simulink model "LAB_03_3_OCT_SIM_EUL"  (R2022b)
settings: Solver=FixedStepAuto  StartTime=0.0  StopTime=100.0  FixedStep=0.1  RelTol=1e-3
values from neighbouring files (symbols this model uses):
  om_x0 = 0.45    [LAB_03_3_OCT_MAT_EUL.m]    (also in LAB_03_3_OCT_MAT_EUL_2_VERIFICATION.m = 6.28318530718; LAB_03_3_OCT_MAT_EUL_DOUBLESPIN.m = 1e-06; LAB_03_3_OCT_MAT_EUL_SPINAXIS.m = 0.1; LAB_03_3_OCT_MAT_EUL_VECT.m)
  om_y0 = 0.52    [LAB_03_3_OCT_MAT_EUL.m]    (also in LAB_03_3_OCT_MAT_EUL_2_VERIFICATION.m = 0; LAB_03_3_OCT_MAT_EUL_DOUBLESPIN.m = 1e-06; LAB_03_3_OCT_MAT_EUL_SPINAXIS.m = 6.28318530718; LAB_03_3_OCT_MAT_EUL_VECT.m)
  om_z0 = 0.55    [LAB_03_3_OCT_MAT_EUL.m]    (also in LAB_03_3_OCT_MAT_EUL_2_VERIFICATION.m = 0; LAB_03_3_OCT_MAT_EUL_DOUBLESPIN.m = 0.02; LAB_03_3_OCT_MAT_EUL_SPINAXIS.m = 0.1; LAB_03_3_OCT_MAT_EUL_VECT.m)
settings Model: Creator=maria  LastModifiedBy=maria

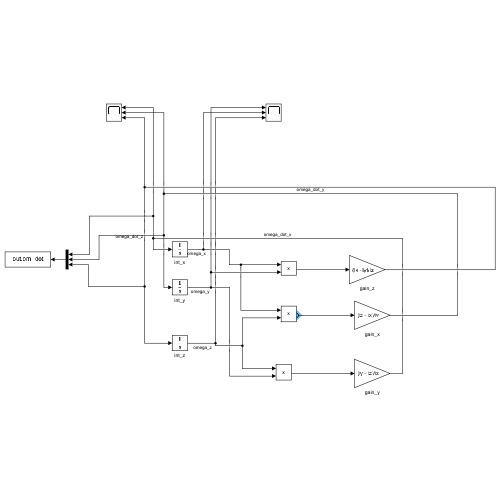
[thumbnail: Simulink's stored preview of the top-level diagram]
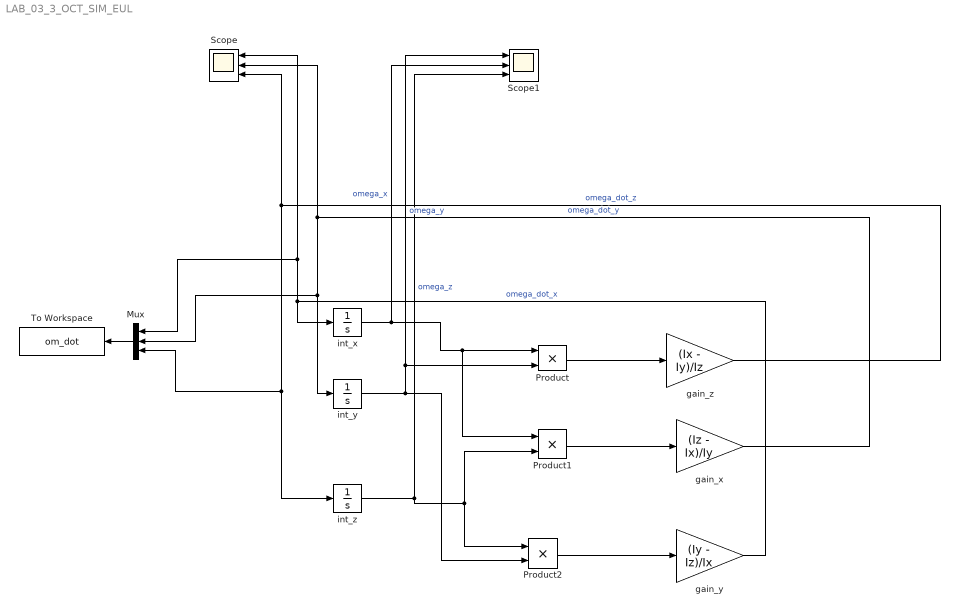
== system LAB_03_3_OCT_SIM_EUL ==
  Mux : Mux  Inputs=3
  Product : Product
  Product1 : Product
  Product2 : Product
  Scope : Scope  NumInputPorts=3
  Scope1 : Scope  NumInputPorts=3
  To Workspace : ToWorkspace  VariableName=om_dot  SaveFormat=Timeseries  SampleTime=-1
  gain_x : Gain  Gain=(Iz - Ix)/Iy
  gain_y : Gain  Gain=(Iy - Iz)/Ix
  gain_z : Gain  Gain=(Ix - Iy)/Iz
  int_x : Integrator  InitialCondition=om_x0
  int_y : Integrator  InitialCondition=om_y0
  int_z : Integrator  InitialCondition=om_z0
  wires:
  int_x/1 -> Scope1/2, Product1/1, Product/1  "omega_x"
  int_y/1 -> Scope1/1, Product/2, Product2/2  "omega_y"
  int_z/1 -> Product2/1, Product1/2, Scope1/3  "omega_z"
  Product2/1 -> gain_y/1
  gain_y/1 -> int_x/1, Mux/1, Scope/1  "omega_dot_x"
  Product/1 -> gain_z/1
  gain_z/1 -> Scope/3, int_z/1, Mux/3  "omega_dot_z"
  Product1/1 -> gain_x/1
  gain_x/1 -> Scope/2, int_y/1, Mux/2  "omega_dot_y"
  Mux/1 -> To Workspace/1
